simulink model "master_thesis_simulink"  (R2022a)
settings: Solver=VariableStepAuto  StartTime=0.0  StopTime=p_0p.time(end)  FixedStep=0.001  RelTol=1e-3
values from neighbouring files (symbols this model uses):
  markers_forearm = [0.00210510253906 -0.143263397217 -0.00798474121094]    [markers_forearm.mat]
  markers_shoulder = [0.010127746582 -0.151647644043 -0.0119686279297]    [markers_shoulder.mat]
undefined symbols (not defined in the file or in its folder): arm, DiscIntNeverNeededParam, Discrete, ekf, kf, LS, m, markers_hand, n, noise, q0, q0_LS, q0_model, sample_Time, selected, state_observer, Time, tSh_0_0Conf, X, Y, Z
libraries: sm_lib x2029, nesl_utility x1553, robotlib x75, ctrlSharedLib x8
(part 3 of 70)

== system master_thesis_simulink/Ros2Matlab/S0_F1_H2/Position_M0 & velocity_M0 computation ==
  p_W : Inport
  v_W : Inport  Port=2
  quat_02W : Inport  Port=3
  " " : Subsystem  TreatAsAtomicUnit=on
  If1 : If
  MATLAB Function3 : MATLAB Function  TreatAsAtomicUnit=on
  Scope10 : Scope
  Terminator3 : Terminator
  p_0' : Outport
  v_0' : Outport  Port=2
  tag scope: isNew=global
  wires:
  v_W/1 -> " "/2(v_W)
  quat_02W/1 -> " "/3(quat_02W)
  p_W/1 -> " "/1(p_W)
  If1/1 -> " "/Action
  MATLAB Function3/1(y) -> [isNew], Scope10/1, If1/1
  [M0_isNew] -> MATLAB Function3/1(M0_isNew)
  If1/2 -> Terminator3/1
  " "/1(p_0') -> p_0'/1
  " "/2(v_0') -> v_0'/1
  [M2_isNew] -> MATLAB Function3/2(M2_isNew)
  [M3_isNew] -> MATLAB Function3/3(M3_isNew)
  [M4_isNew] -> MATLAB Function3/4(M4_isNew)

== system master_thesis_simulink/Ros2Matlab/S0_F1_H2/Subscriber ==
  M0 : Subsystem
  M2 : Subsystem
  M3 : Subsystem
  M4 : Subsystem
  Shoulder_RF : Subsystem
  Terminator : Terminator
  p0_W : Outport
  p2_W : Outport  Port=2
  p3_W : Outport  Port=3
  p4_W : Outport  Port=4
  v0_W : Outport  Port=5
  v2_W : Outport  Port=6
  v3_W : Outport  Port=7
  v4_W : Outport  Port=8
  quat_02W : Outport  Port=9
  pSh_W : Outport  Port=10
  Rp0_W : Outport  Port=11
  Rp2_W : Outport  Port=12
  Rp3_W : Outport  Port=13
  Rp4_W : Outport  Port=14
  Rv0_W : Outport  Port=15
  Rv2_W : Outport  Port=16
  Rv3_W : Outport  Port=17
  Rv4_W : Outport  Port=18
  wires:
  M4/2(v4_W) -> v4_W/1  "v4_W"
  M2/1(p2_W) -> p2_W/1  "p2_W"
  M2/2(v2_W) -> v2_W/1  "v2_W"
  Shoulder_RF/1(pSh_W) -> pSh_W/1
  M0/2(v0_W) -> v0_W/1  "v0_W"
  M3/1(p3_W) -> p3_W/1  "p3_W"
  M3/2(v3_W) -> v3_W/1  "v3_W"
  M0/3(quat_02W) -> quat_02W/1
  M0/1(p0_W) -> p0_W/1  "p0_W"
  M4/1(p4_W) -> p4_W/1  "p4_W"
  Shoulder_RF/2(quat_Sh2W) -> Terminator/1
  M0/4(Rp0_W) -> Rp0_W/1  "Covariance Rp0_W"
  M2/3(Rp2_W) -> Rp2_W/1  "Covariance Rp2_W"
  M3/3(Rp3_W) -> Rp3_W/1  "Covariance Rp3_W"
  M4/3(Rp4_W) -> Rp4_W/1  "Covariance Rp4_W"
  M0/5(Rv0_W) -> Rv0_W/1  "Covariance Rv0_W"
  M2/4(Rv2_W) -> Rv2_W/1  "Covariance Rv2_W"
  M3/4(Rv3_W) -> Rv3_W/1  "Covariance Rv3_W"
  M4/4(Rv4_W) -> Rv4_W/1  "Covariance Rv4_W"

== system master_thesis_simulink/Ros2Matlab/S0_F1_H2/tSh_0 computation ==
  p0_W : Inport
  pSh_W : Inport  Port=2
  quat_02W : Inport  Port=3
  If Action Subsystem1 : Subsystem  TreatAsAtomicUnit=on
  If1 : If
  MATLAB Function3 : MATLAB Function  TreatAsAtomicUnit=on
  Scope10 : Scope
  Terminator3 : Terminator
  tSh_0 : Outport
  wires:
  [Sh_isNew] -> MATLAB Function3/2(Sh_isNew)
  If1/2 -> Terminator3/1
  If Action Subsystem1/1(tSh_0) -> tSh_0/1
  [M0_isNew] -> MATLAB Function3/1(M0_isNew)
  p0_W/1 -> If Action Subsystem1/1(p0_W)
  MATLAB Function3/1(y) -> Scope10/1, If1/1
  If1/1 -> If Action Subsystem1/Action
  pSh_W/1 -> If Action Subsystem1/2(pSh_W)
  quat_02W/1 -> If Action Subsystem1/3(quat_02W)

== system master_thesis_simulink/Ros2Matlab/S0_F2_H2/Position_M0 & velocity_M0 computation ==
  p_W : Inport
  v_W : Inport  Port=2
  quat_02W : Inport  Port=3
  " " : Subsystem  TreatAsAtomicUnit=on
  If1 : If
  MATLAB Function3 : MATLAB Function  TreatAsAtomicUnit=on
  Scope10 : Scope
  Terminator3 : Terminator
  p_0' : Outport
  v_0' : Outport  Port=2
  tag scope: isNew=global
  wires:
  v_W/1 -> " "/2(v_W)
  quat_02W/1 -> " "/3(quat_02W)
  p_W/1 -> " "/1(p_W)
  If1/1 -> " "/Action
  [M1_isNew] -> MATLAB Function3/2(M1_isNew)
  MATLAB Function3/1(y) -> [isNew], Scope10/1, If1/1
  [M0_isNew] -> MATLAB Function3/1(M0_isNew)
  If1/2 -> Terminator3/1
  " "/1(p_0') -> p_0'/1
  " "/2(v_0') -> v_0'/1
  [M2_isNew] -> MATLAB Function3/3(M2_isNew)
  [M3_isNew] -> MATLAB Function3/4(M3_isNew)
  [M4_isNew] -> MATLAB Function3/5(M4_isNew)

== system master_thesis_simulink/Ros2Matlab/S0_F2_H2/Subscriber ==
  M0 : Subsystem
  M1 : Subsystem
  M2 : Subsystem
  M3 : Subsystem
  M4 : Subsystem
  Shoulder_RF : Subsystem
  Terminator : Terminator
  p0_W : Outport
  p1_W : Outport  Port=2
  p2_W : Outport  Port=3
  p3_W : Outport  Port=4
  p4_W : Outport  Port=5
  v0_W : Outport  Port=6
  v1_W : Outport  Port=7
  v2_W : Outport  Port=8
  v3_W : Outport  Port=9
  v4_W : Outport  Port=10
  quat_02W : Outport  Port=11
  pSh_W : Outport  Port=12
  Rp0_W : Outport  Port=13
  Rp1_W : Outport  Port=14
  Rp2_W : Outport  Port=15
  Rp3_W : Outport  Port=16
  Rp4_W : Outport  Port=17
  Rv0_W : Outport  Port=18
  Rv1_W : Outport  Port=19
  Rv2_W : Outport  Port=20
  Rv3_W : Outport  Port=21
  Rv4_W : Outport  Port=22
  wires:
  M4/2(v4_W) -> v4_W/1  "v4_W"
  M2/1(p2_W) -> p2_W/1  "p2_W"
  M2/2(v2_W) -> v2_W/1  "v2_W"
  Shoulder_RF/1(pSh_W) -> pSh_W/1
  M1/1(p1_W) -> p1_W/1  "p1_W"
  M0/2(v0_W) -> v0_W/1  "v0_W"
  M3/1(p3_W) -> p3_W/1  "p3_W"
  M3/2(v3_W) -> v3_W/1  "v3_W"
  M0/3(quat_02W) -> quat_02W/1
  M0/1(p0_W) -> p0_W/1  "p0_W"
  M1/2(v1_W) -> v1_W/1  "v1_W"
  M4/1(p4_W) -> p4_W/1  "p4_W"
  Shoulder_RF/2(quat_Sh2W) -> Terminator/1
  M0/4(Rp0_W) -> Rp0_W/1  "Covariance Rp0_W"
  M1/3(Rp1_W) -> Rp1_W/1  "Covariance Rp1_W"
  M2/3(Rp2_W) -> Rp2_W/1  "Covariance Rp2_W"
  M3/3(Rp3_W) -> Rp3_W/1  "Covariance Rp3_W"
  M4/3(Rp4_W) -> Rp4_W/1  "Covariance Rp4_W"
  M0/5(Rv0_W) -> Rv0_W/1  "Covariance Rv0_W"
  M1/4(Rv1_W) -> Rv1_W/1  "Covariance Rv1_W"
  M2/4(Rv2_W) -> Rv2_W/1  "Covariance Rv2_W"
  M3/4(Rv3_W) -> Rv3_W/1  "Covariance Rv3_W"
  M4/4(Rv4_W) -> Rv4_W/1  "Covariance Rv4_W"

== system master_thesis_simulink/Ros2Matlab/S0_F2_H2/tSh_0 computation ==
  p0_W : Inport
  pSh_W : Inport  Port=2
  quat_02W : Inport  Port=3
  If Action Subsystem1 : Subsystem  TreatAsAtomicUnit=on
  If1 : If
  MATLAB Function3 : MATLAB Function  TreatAsAtomicUnit=on
  Scope10 : Scope
  Terminator3 : Terminator
  tSh_0 : Outport
  wires:
  [Sh_isNew] -> MATLAB Function3/2(Sh_isNew)
  If1/2 -> Terminator3/1
  If Action Subsystem1/1(tSh_0) -> tSh_0/1
  [M0_isNew] -> MATLAB Function3/1(M0_isNew)
  p0_W/1 -> If Action Subsystem1/1(p0_W)
  MATLAB Function3/1(y) -> Scope10/1, If1/1
  If1/1 -> If Action Subsystem1/Action
  pSh_W/1 -> If Action Subsystem1/2(pSh_W)
  quat_02W/1 -> If Action Subsystem1/3(quat_02W)

== system master_thesis_simulink/Ros2Matlab/S1_F0_H2/Position_M0 & velocity_M0 computation ==
  p_W : Inport
  v_W : Inport  Port=2
  quat_02W : Inport  Port=3
  " " : Subsystem  TreatAsAtomicUnit=on
  If1 : If
  MATLAB Function3 : MATLAB Function  TreatAsAtomicUnit=on
  Scope10 : Scope
  Terminator3 : Terminator
  p_0' : Outport
  v_0' : Outport  Port=2
  tag scope: isNew=global
  wires:
  v_W/1 -> " "/2(v_W)
  quat_02W/1 -> " "/3(quat_02W)
  p_W/1 -> " "/1(p_W)
  If1/1 -> " "/Action
  [M1_isNew] -> MATLAB Function3/2(M1_isNew)
  MATLAB Function3/1(y) -> [isNew], Scope10/1, If1/1
  [M0_isNew] -> MATLAB Function3/1(M0_isNew)
  If1/2 -> Terminator3/1
  " "/1(p_0') -> p_0'/1
  " "/2(v_0') -> v_0'/1
  [M3_isNew] -> MATLAB Function3/3(M3_isNew)
  [M4_isNew] -> MATLAB Function3/4(M4_isNew)

== system master_thesis_simulink/Ros2Matlab/S1_F0_H2/Subscriber ==
  M0 : Subsystem
  M1 : Subsystem
  M3 : Subsystem
  M4 : Subsystem
  Shoulder_RF : Subsystem
  Terminator : Terminator
  p0_W : Outport
  p1_W : Outport  Port=2
  p3_W : Outport  Port=3
  p4_W : Outport  Port=4
  v0_W : Outport  Port=5
  v1_W : Outport  Port=6
  v3_W : Outport  Port=7
  v4_W : Outport  Port=8
  quat_02W : Outport  Port=9
  pSh_W : Outport  Port=10
  Rp0_W : Outport  Port=11
  Rp1_W : Outport  Port=12
  Rp3_W : Outport  Port=13
  Rp4_W : Outport  Port=14
  Rv0_W : Outport  Port=15
  Rv1_W : Outport  Port=16
  Rv3_W : Outport  Port=17
  Rv4_W : Outport  Port=18
  wires:
  M4/2(v4_W) -> v4_W/1  "v4_W"
  Shoulder_RF/1(pSh_W) -> pSh_W/1
  M1/1(p1_W) -> p1_W/1  "p1_W"
  M0/2(v0_W) -> v0_W/1  "v0_W"
  M3/1(p3_W) -> p3_W/1  "p3_W"
  M3/2(v3_W) -> v3_W/1  "v3_W"
  M0/3(quat_02W) -> quat_02W/1
  M0/1(p0_W) -> p0_W/1  "p0_W"
  M1/2(v1_W) -> v1_W/1  "v1_W"
  M4/1(p4_W) -> p4_W/1  "p4_W"
  Shoulder_RF/2(quat_Sh2W) -> Terminator/1
  M0/4(Rp0_W) -> Rp0_W/1  "Covariance Rp0_W"
  M1/3(Rp1_W) -> Rp1_W/1  "Covariance Rp1_W"
  M3/3(Rp3_W) -> Rp3_W/1  "Covariance Rp3_W"
  M4/3(Rp4_W) -> Rp4_W/1  "Covariance Rp4_W"
  M0/5(Rv0_W) -> Rv0_W/1  "Covariance Rv0_W"
  M1/4(Rv1_W) -> Rv1_W/1  "Covariance Rv1_W"
  M3/4(Rv3_W) -> Rv3_W/1  "Covariance Rv3_W"
  M4/4(Rv4_W) -> Rv4_W/1  "Covariance Rv4_W"

== system master_thesis_simulink/Ros2Matlab/S1_F0_H2/tSh_0 computation ==
  p0_W : Inport
  pSh_W : Inport  Port=2
  quat_02W : Inport  Port=3
  If Action Subsystem1 : Subsystem  TreatAsAtomicUnit=on
  If1 : If
  MATLAB Function3 : MATLAB Function  TreatAsAtomicUnit=on
  Scope10 : Scope
  Terminator3 : Terminator
  tSh_0 : Outport
  wires:
  [Sh_isNew] -> MATLAB Function3/2(Sh_isNew)
  If1/2 -> Terminator3/1
  If Action Subsystem1/1(tSh_0) -> tSh_0/1
  [M0_isNew] -> MATLAB Function3/1(M0_isNew)
  p0_W/1 -> If Action Subsystem1/1(p0_W)
  MATLAB Function3/1(y) -> Scope10/1, If1/1
  If1/1 -> If Action Subsystem1/Action
  pSh_W/1 -> If Action Subsystem1/2(pSh_W)
  quat_02W/1 -> If Action Subsystem1/3(quat_02W)

== system master_thesis_simulink/Ros2Matlab/S1_F0_H3/Position_M0 & velocity_M0 computation ==
  p_W : Inport
  v_W : Inport  Port=2
  quat_02W : Inport  Port=3
  " " : Subsystem  TreatAsAtomicUnit=on
  If1 : If
  MATLAB Function3 : MATLAB Function  TreatAsAtomicUnit=on
  Scope10 : Scope
  Terminator3 : Terminator
  p_0' : Outport
  v_0' : Outport  Port=2
  tag scope: isNew=global
  wires:
  v_W/1 -> " "/2(v_W)
  quat_02W/1 -> " "/3(quat_02W)
  p_W/1 -> " "/1(p_W)
  If1/1 -> " "/Action
  [M1_isNew] -> MATLAB Function3/2(M1_isNew)
  MATLAB Function3/1(y) -> [isNew], Scope10/1, If1/1
  [M0_isNew] -> MATLAB Function3/1(M0_isNew)
  If1/2 -> Terminator3/1
  " "/1(p_0') -> p_0'/1
  " "/2(v_0') -> v_0'/1
  [M2_isNew] -> MATLAB Function3/3(M2_isNew)
  [M3_isNew] -> MATLAB Function3/4(M3_isNew)
  [M4_isNew] -> MATLAB Function3/5(M4_isNew)

== system master_thesis_simulink/Ros2Matlab/S1_F0_H3/Subscriber ==
  M0 : Subsystem
  M1 : Subsystem
  M2 : Subsystem
  M3 : Subsystem
  M4 : Subsystem
  Shoulder_RF : Subsystem
  Terminator : Terminator
  p0_W : Outport
  p1_W : Outport  Port=2
  p2_W : Outport  Port=3
  p3_W : Outport  Port=4
  p4_W : Outport  Port=5
  v0_W : Outport  Port=6
  v1_W : Outport  Port=7
  v2_W : Outport  Port=8
  v3_W : Outport  Port=9
  v4_W : Outport  Port=10
  quat_02W : Outport  Port=11
  pSh_W : Outport  Port=12
  Rp0_W : Outport  Port=13
  Rp1_W : Outport  Port=14
  Rp2_W : Outport  Port=15
  Rp3_W : Outport  Port=16
  Rp4_W : Outport  Port=17
  Rv0_W : Outport  Port=18
  Rv1_W : Outport  Port=19
  Rv2_W : Outport  Port=20
  Rv3_W : Outport  Port=21
  Rv4_W : Outport  Port=22
  wires:
  M4/2(v4_W) -> v4_W/1  "v4_W"
  M2/1(p2_W) -> p2_W/1  "p2_W"
  M2/2(v2_W) -> v2_W/1  "v2_W"
  Shoulder_RF/1(pSh_W) -> pSh_W/1
  M1/1(p1_W) -> p1_W/1  "p1_W"
  M0/2(v0_W) -> v0_W/1  "v0_W"
  M3/1(p3_W) -> p3_W/1  "p3_W"
  M3/2(v3_W) -> v3_W/1  "v3_W"
  M0/3(quat_02W) -> quat_02W/1
  M0/1(p0_W) -> p0_W/1  "p0_W"
  M1/2(v1_W) -> v1_W/1  "v1_W"
  M4/1(p4_W) -> p4_W/1  "p4_W"
  Shoulder_RF/2(quat_Sh2W) -> Terminator/1
  M0/4(Rp0_W) -> Rp0_W/1  "Covariance Rp0_W"
  M1/3(Rp1_W) -> Rp1_W/1  "Covariance Rp1_W"
  M2/3(Rp2_W) -> Rp2_W/1  "Covariance Rp2_W"
  M3/3(Rp3_W) -> Rp3_W/1  "Covariance Rp3_W"
  M4/3(Rp4_W) -> Rp4_W/1  "Covariance Rp4_W"
  M0/5(Rv0_W) -> Rv0_W/1  "Covariance Rv0_W"
  M1/4(Rv1_W) -> Rv1_W/1  "Covariance Rv1_W"
  M2/4(Rv2_W) -> Rv2_W/1  "Covariance Rv2_W"
  M3/4(Rv3_W) -> Rv3_W/1  "Covariance Rv3_W"
  M4/4(Rv4_W) -> Rv4_W/1  "Covariance Rv4_W"

== system master_thesis_simulink/Ros2Matlab/S1_F0_H3/tSh_0 computation ==
  p0_W : Inport
  pSh_W : Inport  Port=2
  quat_02W : Inport  Port=3
  If Action Subsystem1 : Subsystem  TreatAsAtomicUnit=on
  If1 : If
  MATLAB Function3 : MATLAB Function  TreatAsAtomicUnit=on
  Scope10 : Scope
  Terminator3 : Terminator
  tSh_0 : Outport
  wires:
  [Sh_isNew] -> MATLAB Function3/2(Sh_isNew)
  If1/2 -> Terminator3/1
  If Action Subsystem1/1(tSh_0) -> tSh_0/1
  [M0_isNew] -> MATLAB Function3/1(M0_isNew)
  p0_W/1 -> If Action Subsystem1/1(p0_W)
  MATLAB Function3/1(y) -> Scope10/1, If1/1
  If1/1 -> If Action Subsystem1/Action
  pSh_W/1 -> If Action Subsystem1/2(pSh_W)
  quat_02W/1 -> If Action Subsystem1/3(quat_02W)

== system master_thesis_simulink/Ros2Matlab/S1_F1_H2/Position_M0 & velocity_M0 computation ==
  p_W : Inport
  v_W : Inport  Port=2
  quat_02W : Inport  Port=3
  " " : Subsystem  TreatAsAtomicUnit=on
  If1 : If
  MATLAB Function3 : MATLAB Function  TreatAsAtomicUnit=on
  Scope10 : Scope
  Terminator3 : Terminator
  p_0' : Outport
  v_0' : Outport  Port=2
  tag scope: isNew=global
  wires:
  v_W/1 -> " "/2(v_W)
  quat_02W/1 -> " "/3(quat_02W)
  p_W/1 -> " "/1(p_W)
  If1/1 -> " "/Action
  [M1_isNew] -> MATLAB Function3/2(M1_isNew)
  MATLAB Function3/1(y) -> [isNew], Scope10/1, If1/1
  [M0_isNew] -> MATLAB Function3/1(M0_isNew)
  If1/2 -> Terminator3/1
  " "/1(p_0') -> p_0'/1
  " "/2(v_0') -> v_0'/1
  [M2_isNew] -> MATLAB Function3/3(M2_isNew)
  [M3_isNew] -> MATLAB Function3/4(M3_isNew)
  [M4_isNew] -> MATLAB Function3/5(M4_isNew)

== system master_thesis_simulink/Ros2Matlab/S1_F1_H2/Subscriber ==
  M0 : Subsystem
  M1 : Subsystem
  M2 : Subsystem
  M3 : Subsystem
  M4 : Subsystem
  Shoulder_RF : Subsystem
  Terminator : Terminator
  p0_W : Outport
  p1_W : Outport  Port=2
  p2_W : Outport  Port=3
  p3_W : Outport  Port=4
  p4_W : Outport  Port=5
  v0_W : Outport  Port=6
  v1_W : Outport  Port=7
  v2_W : Outport  Port=8
  v3_W : Outport  Port=9
  v4_W : Outport  Port=10
  quat_02W : Outport  Port=11
  pSh_W : Outport  Port=12
  Rp0_W : Outport  Port=13
  Rp1_W : Outport  Port=14
  Rp2_W : Outport  Port=15
  Rp3_W : Outport  Port=16
  Rp4_W : Outport  Port=17
  Rv0_W : Outport  Port=18
  Rv1_W : Outport  Port=19
  Rv2_W : Outport  Port=20
  Rv3_W : Outport  Port=21
  Rv4_W : Outport  Port=22
  wires:
  M4/2(v4_W) -> v4_W/1  "v4_W"
  M2/1(p2_W) -> p2_W/1  "p2_W"
  M2/2(v2_W) -> v2_W/1  "v2_W"
  Shoulder_RF/1(pSh_W) -> pSh_W/1
  M1/1(p1_W) -> p1_W/1  "p1_W"
  M0/2(v0_W) -> v0_W/1  "v0_W"
  M3/1(p3_W) -> p3_W/1  "p3_W"
  M3/2(v3_W) -> v3_W/1  "v3_W"
  M0/3(quat_02W) -> quat_02W/1
  M0/1(p0_W) -> p0_W/1  "p0_W"
  M1/2(v1_W) -> v1_W/1  "v1_W"
  M4/1(p4_W) -> p4_W/1  "p4_W"
  Shoulder_RF/2(quat_Sh2W) -> Terminator/1
  M0/4(Rp0_W) -> Rp0_W/1  "Covariance Rp0_W"
  M1/3(Rp1_W) -> Rp1_W/1  "Covariance Rp1_W"
  M2/3(Rp2_W) -> Rp2_W/1  "Covariance Rp2_W"
  M3/3(Rp3_W) -> Rp3_W/1  "Covariance Rp3_W"
  M4/3(Rp4_W) -> Rp4_W/1  "Covariance Rp4_W"
  M0/5(Rv0_W) -> Rv0_W/1  "Covariance Rv0_W"
  M1/4(Rv1_W) -> Rv1_W/1  "Covariance Rv1_W"
  M2/4(Rv2_W) -> Rv2_W/1  "Covariance Rv2_W"
  M3/4(Rv3_W) -> Rv3_W/1  "Covariance Rv3_W"
  M4/4(Rv4_W) -> Rv4_W/1  "Covariance Rv4_W"

== system master_thesis_simulink/Ros2Matlab/S1_F1_H2/tSh_0 computation ==
  p0_W : Inport
  pSh_W : Inport  Port=2
  quat_02W : Inport  Port=3
  If Action Subsystem1 : Subsystem  TreatAsAtomicUnit=on
  If1 : If
  MATLAB Function3 : MATLAB Function  TreatAsAtomicUnit=on
  Scope10 : Scope
  Terminator3 : Terminator
  tSh_0 : Outport
  wires:
  [Sh_isNew] -> MATLAB Function3/2(Sh_isNew)
  If1/2 -> Terminator3/1
  If Action Subsystem1/1(tSh_0) -> tSh_0/1
  [M0_isNew] -> MATLAB Function3/1(M0_isNew)
  p0_W/1 -> If Action Subsystem1/1(p0_W)
  MATLAB Function3/1(y) -> Scope10/1, If1/1
  If1/1 -> If Action Subsystem1/Action
  pSh_W/1 -> If Action Subsystem1/2(pSh_W)
  quat_02W/1 -> If Action Subsystem1/3(quat_02W)

== system master_thesis_simulink/Ros2Matlab/S1_F2_H2/Position_M0 & velocity_M0 computation ==
  p_W : Inport
  v_W : Inport  Port=2
  quat_02W : Inport  Port=3
  " " : Subsystem  TreatAsAtomicUnit=on
  If1 : If
  MATLAB Function3 : MATLAB Function  TreatAsAtomicUnit=on
  Scope10 : Scope
  Terminator3 : Terminator
  p_0' : Outport
  v_0' : Outport  Port=2
  tag scope: isNew=global
  wires:
  [M4_isNew] -> MATLAB Function3/5(M4_isNew)
  [M3_isNew] -> MATLAB Function3/4(M3_isNew)
  [M2_isNew] -> MATLAB Function3/3(M2_isNew)
  " "/2(v_0') -> v_0'/1
  " "/1(p_0') -> p_0'/1
  If1/2 -> Terminator3/1
  [M0_isNew] -> MATLAB Function3/1(M0_isNew)
  MATLAB Function3/1(y) -> If1/1, Scope10/1, [isNew]
  [M1_isNew] -> MATLAB Function3/2(M1_isNew)
  If1/1 -> " "/Action
  p_W/1 -> " "/1(p_W)
  quat_02W/1 -> " "/3(quat_02W)
  v_W/1 -> " "/2(v_W)
  [M5_isNew] -> MATLAB Function3/6(M5_isNew)

== system master_thesis_simulink/Ros2Matlab/S1_F2_H2/Subscriber ==
  M0 : Subsystem
  M1 : Subsystem
  M2 : Subsystem
  M3 : Subsystem
  M4 : Subsystem
  M5 : Subsystem
  Shoulder_RF : Subsystem
  Terminator : Terminator
  p0_W : Outport
  p1_W : Outport  Port=2
  p2_W : Outport  Port=3
  p3_W : Outport  Port=4
  p4_W : Outport  Port=5
  v0_W : Outport  Port=6
  v1_W : Outport  Port=7
  v2_W : Outport  Port=8
  v3_W : Outport  Port=9
  v4_W : Outport  Port=10
  quat_02W : Outport  Port=11
  pSh_W : Outport  Port=12
  Rp0_W : Outport  Port=13
  Rp1_W : Outport  Port=14
  Rp2_W : Outport  Port=15
  Rp3_W : Outport  Port=16
  Rp4_W : Outport  Port=17
  Rv0_W : Outport  Port=18
  Rv1_W : Outport  Port=19
  Rv2_W : Outport  Port=20
  Rv3_W : Outport  Port=21
  Rv4_W : Outport  Port=22
  p5_W : Outport  Port=23
  v5_W : Outport  Port=24
  Rp5_W : Outport  Port=25
  Rv5_W : Outport  Port=26
  wires:
  M4/4(Rv4_W) -> Rv4_W/1  "Covariance Rv4_W"
  M3/4(Rv3_W) -> Rv3_W/1  "Covariance Rv3_W"
  M2/4(Rv2_W) -> Rv2_W/1  "Covariance Rv2_W"
  M1/4(Rv1_W) -> Rv1_W/1  "Covariance Rv1_W"
  M0/5(Rv0_W) -> Rv0_W/1  "Covariance Rv0_W"
  M4/3(Rp4_W) -> Rp4_W/1  "Covariance Rp4_W"
  M3/3(Rp3_W) -> Rp3_W/1  "Covariance Rp3_W"
  M2/3(Rp2_W) -> Rp2_W/1  "Covariance Rp2_W"
  M1/3(Rp1_W) -> Rp1_W/1  "Covariance Rp1_W"
  M0/4(Rp0_W) -> Rp0_W/1  "Covariance Rp0_W"
  Shoulder_RF/2(quat_Sh2W) -> Terminator/1
  M4/1(p4_W) -> p4_W/1  "p4_W"
  M1/2(v1_W) -> v1_W/1  "v1_W"
  M0/1(p0_W) -> p0_W/1  "p0_W"
  M0/3(quat_02W) -> quat_02W/1
  M3/2(v3_W) -> v3_W/1  "v3_W"
  M3/1(p3_W) -> p3_W/1  "p3_W"
  M0/2(v0_W) -> v0_W/1  "v0_W"
  M1/1(p1_W) -> p1_W/1  "p1_W"
  Shoulder_RF/1(pSh_W) -> pSh_W/1
  M2/2(v2_W) -> v2_W/1  "v2_W"
  M2/1(p2_W) -> p2_W/1  "p2_W"
  M4/2(v4_W) -> v4_W/1  "v4_W"
  M5/1(p2_W) -> p5_W/1  "p2_W"
  M5/2(v2_W) -> v5_W/1  "v2_W"
  M5/3(Rp2_W) -> Rp5_W/1  "Covariance Rp2_W"
  M5/4(Rv2_W) -> Rv5_W/1  "Covariance Rv2_W"

== system master_thesis_simulink/Ros2Matlab/S1_F2_H2/tSh_0 computation ==
  p0_W : Inport
  pSh_W : Inport  Port=2
  quat_02W : Inport  Port=3
  If Action Subsystem1 : Subsystem  TreatAsAtomicUnit=on
  If1 : If
  MATLAB Function3 : MATLAB Function  TreatAsAtomicUnit=on
  Scope10 : Scope
  Terminator3 : Terminator
  tSh_0 : Outport
  wires:
  quat_02W/1 -> If Action Subsystem1/3(quat_02W)
  pSh_W/1 -> If Action Subsystem1/2(pSh_W)
  If1/1 -> If Action Subsystem1/Action
  MATLAB Function3/1(y) -> If1/1, Scope10/1
  p0_W/1 -> If Action Subsystem1/1(p0_W)
  [M0_isNew] -> MATLAB Function3/1(M0_isNew)
  If Action Subsystem1/1(tSh_0) -> tSh_0/1
  If1/2 -> Terminator3/1
  [Sh_isNew] -> MATLAB Function3/2(Sh_isNew)

== system master_thesis_simulink/Ros2Matlab/S2_F0_H2/Position_M0 & velocity_M0 computation ==
  p_W : Inport
  v_W : Inport  Port=2
  quat_02W : Inport  Port=3
  " " : Subsystem  TreatAsAtomicUnit=on
  If1 : If
  MATLAB Function3 : MATLAB Function  TreatAsAtomicUnit=on
  Scope10 : Scope
  Terminator3 : Terminator
  p_0' : Outport
  v_0' : Outport  Port=2
  tag scope: isNew=global
  wires:
  v_W/1 -> " "/2(v_W)
  quat_02W/1 -> " "/3(quat_02W)
  p_W/1 -> " "/1(p_W)
  If1/1 -> " "/Action
  [M1_isNew] -> MATLAB Function3/2(M1_isNew)
  MATLAB Function3/1(y) -> [isNew], Scope10/1, If1/1
  [M0_isNew] -> MATLAB Function3/1(M0_isNew)
  If1/2 -> Terminator3/1
  " "/1(p_0') -> p_0'/1
  " "/2(v_0') -> v_0'/1
  [M2_isNew] -> MATLAB Function3/3(M2_isNew)
  [M3_isNew] -> MATLAB Function3/4(M3_isNew)
  [M4_isNew] -> MATLAB Function3/5(M4_isNew)

== system master_thesis_simulink/Ros2Matlab/S2_F0_H2/Subscriber ==
  M0 : Subsystem
  M1 : Subsystem
  M2 : Subsystem
  M3 : Subsystem
  M4 : Subsystem
  Shoulder_RF : Subsystem
  Terminator : Terminator
  p0_W : Outport
  p1_W : Outport  Port=2
  p2_W : Outport  Port=3
  p3_W : Outport  Port=4
  p4_W : Outport  Port=5
  v0_W : Outport  Port=6
  v1_W : Outport  Port=7
  v2_W : Outport  Port=8
  v3_W : Outport  Port=9
  v4_W : Outport  Port=10
  quat_02W : Outport  Port=11
  pSh_W : Outport  Port=12
  Rp0_W : Outport  Port=13
  Rp1_W : Outport  Port=14
  Rp2_W : Outport  Port=15
  Rp3_W : Outport  Port=16
  Rp4_W : Outport  Port=17
  Rv0_W : Outport  Port=18
  Rv1_W : Outport  Port=19
  Rv2_W : Outport  Port=20
  Rv3_W : Outport  Port=21
  Rv4_W : Outport  Port=22
  wires:
  M4/2(v4_W) -> v4_W/1  "v4_W"
  M2/1(p2_W) -> p2_W/1  "p2_W"
  M2/2(v2_W) -> v2_W/1  "v2_W"
  Shoulder_RF/1(pSh_W) -> pSh_W/1
  M1/1(p1_W) -> p1_W/1  "p1_W"
  M0/2(v0_W) -> v0_W/1  "v0_W"
  M3/1(p3_W) -> p3_W/1  "p3_W"
  M3/2(v3_W) -> v3_W/1  "v3_W"
  M0/3(quat_02W) -> quat_02W/1
  M0/1(p0_W) -> p0_W/1  "p0_W"
  M1/2(v1_W) -> v1_W/1  "v1_W"
  M4/1(p4_W) -> p4_W/1  "p4_W"
  Shoulder_RF/2(quat_Sh2W) -> Terminator/1
  M0/4(Rp0_W) -> Rp0_W/1  "Covariance Rp0_W"
  M1/3(Rp1_W) -> Rp1_W/1  "Covariance Rp1_W"
  M2/3(Rp2_W) -> Rp2_W/1  "Covariance Rp2_W"
  M3/3(Rp3_W) -> Rp3_W/1  "Covariance Rp3_W"
  M4/3(Rp4_W) -> Rp4_W/1  "Covariance Rp4_W"
  M0/5(Rv0_W) -> Rv0_W/1  "Covariance Rv0_W"
  M1/4(Rv1_W) -> Rv1_W/1  "Covariance Rv1_W"
  M2/4(Rv2_W) -> Rv2_W/1  "Covariance Rv2_W"
  M3/4(Rv3_W) -> Rv3_W/1  "Covariance Rv3_W"
  M4/4(Rv4_W) -> Rv4_W/1  "Covariance Rv4_W"

== system master_thesis_simulink/Ros2Matlab/S2_F0_H2/tSh_0 computation ==
  p0_W : Inport
  pSh_W : Inport  Port=2
  quat_02W : Inport  Port=3
  If Action Subsystem1 : Subsystem  TreatAsAtomicUnit=on
  If1 : If
  MATLAB Function3 : MATLAB Function  TreatAsAtomicUnit=on
  Scope10 : Scope
  Terminator3 : Terminator
  tSh_0 : Outport
  wires:
  [Sh_isNew] -> MATLAB Function3/2(Sh_isNew)
  If1/2 -> Terminator3/1
  If Action Subsystem1/1(tSh_0) -> tSh_0/1
  [M0_isNew] -> MATLAB Function3/1(M0_isNew)
  p0_W/1 -> If Action Subsystem1/1(p0_W)
  MATLAB Function3/1(y) -> Scope10/1, If1/1
  If1/1 -> If Action Subsystem1/Action
  pSh_W/1 -> If Action Subsystem1/2(pSh_W)
  quat_02W/1 -> If Action Subsystem1/3(quat_02W)

== system master_thesis_simulink/System/Human arm/Elbow_joint ==
  q ref 4 : Inport
  PS-Simulink Converter1 : nesl_utility/PS-Simulink Converter  PhysicalDomain=network_engine_domain  SubClassName=ps_output  LeftPortType=input  RightPortType=output  PseudoPeriodic=off  Frequencies=[]  VectorFormat=inherit  Unit=inherit  AffineConversion=off
      settings: SourceProductBaseCode=SS,PW,VE
  PS-Simulink Converter6 : nesl_utility/PS-Simulink Converter  PhysicalDomain=network_engine_domain  SubClassName=ps_output  LeftPortType=input  RightPortType=output  PseudoPeriodic=off  Frequencies=[]  VectorFormat=inherit  Unit=inherit  AffineConversion=off
      settings: SourceProductBaseCode=SS,PW,VE
  c1 : nesl_utility/Simulink-PS Converter  PhysicalDomain=network_engine_domain  SubClassName=ps_input  LeftPortType=input  RightPortType=output  PseudoPeriodic=off  Frequencies=[]  NoiseDistribution=none  NoiseParameters=[]  Unit=1  AffineConversion=off  FilteringAndDerivatives=filter  SimscapeFilterOrder=2  InputFilterTimeConstant=0.001  UdotUserProvided=0
      settings: SourceProductBaseCode=SS,PW,VE
  jRightElbow_rotx : sm_lib/Joints/Revolute Joint  JointMode=Normal  SenseConstraintForce=off  SenseConstraintForceX=off  SenseConstraintForceY=off  SenseConstraintForceZ=off  SenseConstraintTorque=off  SenseConstraintTorqueX=off  SenseConstraintTorqueY=off  SenseConstraintTorqueZ=off  SenseTotalForce=off  SenseTotalForceX=off  SenseTotalForceY=off  SenseTotalForceZ=off  SenseTotalTorque=off  SenseTotalTorqueX=off  SenseTotalTorqueY=off  SenseTotalTorqueZ=off  CompositeWrenchDir=FollowerOnBase  CompositeWrenchFrame=BaseFrame  EquilibriumPosition=0  EquilibriumPositionUnits=deg  SpringStiffness=0  SpringStiffnessUnits=N*m/deg  DampingCoefficient=0.1  DampingCoefficientUnits=kg*m^2/(rad*s)  TorqueActuationMode=ComputedTorque  MotionActuationMode=InputMotion  SensePosition=on  SenseVelocity=on  SenseAcceleration=off  SenseTorqueForce=off  SenseLowerLimitTorqueForce=off  SenseUpperLimitTorqueForce=off  LowerLimitSpecify=on  LowerLimitBound=-3/4*pi  LowerLimitBoundUnits=rad  LowerLimitStiffness=1e4  LowerLimitStiffnessUnits=N*m/deg  LowerLimitDamping=10  LowerLimitDampingUnits=N*m/(deg/s)  LowerLimitTransitionRegionWidth=0.1  LowerLimitTransitionRegionWidthUnits=deg  UpperLimitSpecify=on  UpperLimitBound=0  UpperLimitBoundUnits=rad  UpperLimitStiffness=1e4  UpperLimitStiffnessUnits=N*m/deg  UpperLimitDamping=10  UpperLimitDampingUnits=N*m/(deg/s)  UpperLimitTransitionRegionWidth=0.1  UpperLimitTransitionRegionWidthUnits=deg  PositionTargetSpecify=off  PositionTargetPriority=High  PositionTargetValue=q0(4)  PositionTargetValueUnits=rad  VelocityTargetSpecify=off  VelocityTargetPriority=High  VelocityTargetValue=0  VelocityTargetValueUnits=deg/s
  B_elbow : PMIOPort  Side=Right
  F_shoulder : PMIOPort  Port=2  Side=Left
  tag scope: q4=global, qdot4=global
  wires:
  PS-Simulink Converter6/1 -> [q4]
  PS-Simulink Converter1/1 -> [qdot4]
  q ref 4/1 -> c1/1
  connections:
  jRightElbow_rotx/RConn2 -- PS-Simulink Converter6/LConn1
  PS-Simulink Converter1/LConn1 -- jRightElbow_rotx/RConn3
  ?
  ?
  F_shoulder/RConn1 -- jRightElbow_rotx/LConn1
  jRightElbow_rotx/RConn1 -- B_elbow/RConn1
  c1/RConn1 -- jRightElbow_rotx/LConn2

== system master_thesis_simulink/System/Human arm/Markers ==
  M1 : Subsystem
  W : PMIOPort  Side=Left
  R : PMIOPort  Port=2  Side=Left
  tag scope: p=global, pdot=global
  wires:
  M1/1(p_1) -> [p]
  M1/2(pdot_1) -> [pdot]
  connections:
  R/RConn1 -- M1/LConn2
  W/RConn1 -- M1/LConn1

== system master_thesis_simulink/System/Human arm/RightForeArm ==
  B_elbow__Eend : sm_lib/Frames and Transforms/Rigid Transform  TranslationMethod=Cartesian  TranslationStandardOffset=0  TranslationLengthUnit=m  TranslationStandardAxis=+Z  TranslationCartesianOffset=[0, -arm.forearm.length, 0]  TranslationROffset=0  TranslationROffsetUnits=m  TranslationZOffset=0  TranslationZOffsetUnits=m  TranslationThetaOffset=0  TranslationThetaOffsetUnits=deg  RotationMethod=None  RotationAngleUnits=deg  RotationStandardAxis=+Z  RotationAngle=0.0  RotationArbitraryAxis=[0 0 1]  FollAlignAxisA=+X  BaseAlignAxisA=+Y  FollAlignAxisB=+Y  BaseAlignAxisB=+Z  RotationSequenceAxes=BaseAxes  RotationSequence=XYZ  RotationSequenceAngles=[0, 0, 0]  RotationSequenceAnglesUnits=rad  RotationMatrix=[1 0 0; 0 1 0; 0 0 1]
  B_elbow_setting : sm_lib/Frames and Transforms/Rigid Transform  TranslationMethod=Cartesian  TranslationStandardOffset=0  TranslationLengthUnit=m  TranslationStandardAxis=+Z  TranslationCartesianOffset=[0, arm.forearm.length/2, 0]  TranslationROffset=0  TranslationROffsetUnits=m  TranslationZOffset=0  TranslationZOffsetUnits=m  TranslationThetaOffset=0  TranslationThetaOffsetUnits=deg  RotationMethod=None  RotationAngleUnits=rad  RotationStandardAxis=+Z  RotationAngle=pi/2  RotationArbitraryAxis=[1 0 0]  FollAlignAxisA=+X  BaseAlignAxisA=+Y  FollAlignAxisB=+Y  BaseAlignAxisB=+Z  RotationSequenceAxes=BaseAxes  RotationSequence=XYZ  RotationSequenceAngles=[pi/2, 0, 0]  RotationSequenceAnglesUnits=rad  RotationMatrix=[1 0 0; 0 1 0; 0 0 1]
  ForeArm : sm_lib/Body Elements/Cylindrical Solid  GraphicAmbientColor=[0.15 0.15 0.15 1.0]  BasedOnType=Density  CenterOfMass=[0, 0, 0]  CenterOfMassUnits=m  GraphicDiffuseColor=[0.1, 0.1, 0.1]  CylinderLength=arm.forearm.length  CylinderLengthUnits=m  CylinderRadius=arm.forearm.radius  CylinderRadiusUnits=m  Density=1000  DensityUnits=kg/m^3  DoExposeReferenceFrame=on  GraphicEmissiveColor=[0.0 0.0 0.0 1.0]  ExportEntireGeometry=off  SerializedFrames=<Frames/>  MarkerShape=Sphere  MarkerSize=10  GraphicType=FromGeometry  InertiaType=CalculateFromGeometry  Mass=0  MassUnits=kg  MomentsOfInertia=[0, 0, 0]  MomentsOfInertiaUnits=kg*m^2  GraphicOpacity=1  ProductsOfInertia=[0, 0, 0]  ProductsOfInertiaUnits=kg*m^2  GraphicShininess=75  GraphicSpecularColor=[0.5 0.5 0.5 1.0]  GraphicVisPropType=SimpleVisualProperties
  Inertia1 : sm_lib/Body Elements/Inertia  InertiaType=Custom  Mass=arm.forearm.mass  MassUnits=kg  CenterOfMass=[0 0 0]  CenterOfMassUnits=m  MomentsOfInertia=arm.forearm.moment_inertia  MomentsOfInertiaUnits=kg*m^2  ProductsOfInertia=[0 0 0]  ProductsOfInertiaUnits=kg*m^2  GraphicType=None  MarkerShape=Inertia  MarkerSize=20  GraphicVisPropType=SimpleVisualProperties  GraphicDiffuseColor=[0.5 0.5 0.5]  GraphicSpecularColor=[0.5 0.5 0.5 1.0]  GraphicAmbientColor=[0.15 0.15 0.15 1.0]  GraphicEmissiveColor=[0.0 0.0 0.0 1.0]  GraphicShininess=75  GraphicOpacity=1.0
  Mux : Mux  Inputs=3
  PS-Simulink Converter : nesl_utility/PS-Simulink Converter  PhysicalDomain=network_engine_domain  SubClassName=ps_output  LeftPortType=input  RightPortType=output  PseudoPeriodic=off  Frequencies=[]  VectorFormat=inherit  Unit=inherit  AffineConversion=off
      settings: SourceProductBaseCode=SS,PW,VE
  PS-Simulink Converter1 : nesl_utility/PS-Simulink Converter  PhysicalDomain=network_engine_domain  SubClassName=ps_output  LeftPortType=input  RightPortType=output  PseudoPeriodic=off  Frequencies=[]  VectorFormat=inherit  Unit=inherit  AffineConversion=off
      settings: SourceProductBaseCode=SS,PW,VE
  PS-Simulink Converter2 : nesl_utility/PS-Simulink Converter  PhysicalDomain=network_engine_domain  SubClassName=ps_output  LeftPortType=input  RightPortType=output  PseudoPeriodic=off  Frequencies=[]  VectorFormat=inherit  Unit=inherit  AffineConversion=off
      settings: SourceProductBaseCode=SS,PW,VE
  Reference Frame : sm_lib/Frames and Transforms/Reference Frame
  RighForeArm_rot : sm_lib/Frames and Transforms/Rigid Transform  TranslationMethod=None  TranslationStandardOffset=0  TranslationLengthUnit=m  TranslationStandardAxis=+Z  TranslationCartesianOffset=[0 0 0]  TranslationROffset=0  TranslationROffsetUnits=m  TranslationZOffset=0  TranslationZOffsetUnits=m  TranslationThetaOffset=0  TranslationThetaOffsetUnits=deg  RotationMethod=ArbitraryAxis  RotationAngleUnits=rad  RotationStandardAxis=+Z  RotationAngle=pi/2  RotationArbitraryAxis=[1 0 0]  FollAlignAxisA=+X  BaseAlignAxisA=+Y  FollAlignAxisB=+Y  BaseAlignAxisB=+Z  RotationSequenceAxes=BaseAxes  RotationSequence=XYZ  RotationSequenceAngles=[pi/2, 0, 0]  RotationSequenceAnglesUnits=rad  RotationMatrix=[1 0 0; 0 1 0; 0 0 1]
  Scope : Scope
  Transform Sensor : sm_lib/Frames and Transforms/Transform Sensor  MeasurementFrame=World  SenseAngle=off  SenseAxis=off  SenseAngle1=off  SenseAngle2=off  SenseAngle3=off  SenseQ=off  SenseR=off  SenseOmegaX=off  SenseOmegaY=off  SenseOmegaZ=off  SenseOmega1=off  SenseOmega2=off  SenseOmega3=off  SenseQDot=off  SenseRDot=off  SenseAlphaX=off  SenseAlphaY=off  SenseAlphaZ=off  SenseAlpha1=off  SenseAlpha2=off  SenseAlpha3=off  SenseQDDot=off  SenseRDDot=off  SenseX=on  SenseY=on  SenseZ=on  SenseRad=off  SenseAzim=off  SenseDist=off  SenseInc=off  SenseXDot=off  SenseYDot=off  SenseZDot=off  SenseRadDot=off  SenseAzimDot=off  SenseDistDot=off  SenseIncDot=off  SenseXDDot=off  SenseYDDot=off  SenseZDDot=off  SenseRadDDot=off  SenseAzimDDot=off  SenseDistDDot=off  SenseIncDDot=off
  B_elbow : PMIOPort  Side=Left
  F_elbow : PMIOPort  Port=2  Side=Right
  W : PMIOPort  Port=3  Side=Left
  wires:
  PS-Simulink Converter2/1 -> Mux/3  "elbow_posz"
  Mux/1 -> Scope/1
  PS-Simulink Converter1/1 -> Mux/2  "elbow_posy"
  PS-Simulink Converter/1 -> Mux/1  "elbow_posx"
  connections:
  B_elbow__Eend/RConn1 -- F_elbow/RConn1
  B_elbow__Eend/LConn1 -- B_elbow_setting/RConn1 -- B_elbow/RConn1 -- Transform Sensor/RConn1
  PS-Simulink Converter/LConn1 -- Transform Sensor/RConn2
  PS-Simulink Converter1/LConn1 -- Transform Sensor/RConn3
  PS-Simulink Converter2/LConn1 -- Transform Sensor/RConn4
  ForeArm/RConn1 -- RighForeArm_rot/LConn1
  W/RConn1 -- Transform Sensor/LConn1
  RighForeArm_rot/RConn1 -- Reference Frame/RConn1 -- Inertia1/RConn1 -- B_elbow_setting/LConn1

== system master_thesis_simulink/System/Human arm/RightHand ==
  B_wrist__setting : sm_lib/Frames and Transforms/Rigid Transform  TranslationMethod=Cartesian  TranslationStandardOffset=0  TranslationLengthUnit=m  TranslationStandardAxis=+Z  TranslationCartesianOffset=[0, arm.hand.dimensions(2)/2, 0]  TranslationROffset=0  TranslationROffsetUnits=m  TranslationZOffset=0  TranslationZOffsetUnits=m  TranslationThetaOffset=0  TranslationThetaOffsetUnits=deg  RotationMethod=None  RotationAngleUnits=deg  RotationStandardAxis=+Z  RotationAngle=0.0  RotationArbitraryAxis=[0 0 1]  FollAlignAxisA=+X  BaseAlignAxisA=+Y  FollAlignAxisB=+Y  BaseAlignAxisB=+Z  RotationSequenceAxes=BaseAxes  RotationSequence=XYZ  RotationSequenceAngles=[0, 0, 0]  RotationSequenceAnglesUnits=rad  RotationMatrix=[1 0 0; 0 1 0; 0 0 1]
  Hand : sm_lib/Body Elements/Brick Solid  GraphicAmbientColor=[0.15 0.15 0.15 1.0]  BasedOnType=Density  BrickDimensions=arm.hand.dimensions  BrickDimensionUnits=m  CenterOfMass=[0, 0, 0]  CenterOfMassUnits=m  GraphicDiffuseColor=[0.1, 0.1, 0.1]  Density=1000  DensityUnits=kg/m^3  DoExposeReferenceFrame=on  GraphicEmissiveColor=[0.0 0.0 0.0 1.0]  ExportEntireGeometry=off  SerializedFrames=<Frames/>  MarkerShape=Sphere  MarkerSize=10  GraphicType=FromGeometry  InertiaType=CalculateFromGeometry  Mass=0  MassUnits=kg  MomentsOfInertia=[0, 0, 0]  MomentsOfInertiaUnits=kg*m^2  GraphicOpacity=1  ProductsOfInertia=[0, 0, 0]  ProductsOfInertiaUnits=kg*m^2  GraphicShininess=75  GraphicSpecularColor=[0.5 0.5 0.5 1.0]  GraphicVisPropType=SimpleVisualProperties
  Inertia : sm_lib/Body Elements/Inertia  InertiaType=Custom  Mass=arm.hand.mass  MassUnits=kg  CenterOfMass=[0, 0, 0]  CenterOfMassUnits=m  MomentsOfInertia=arm.hand.moment_inertia  MomentsOfInertiaUnits=kg*m^2  ProductsOfInertia=[0, 0, 0]  ProductsOfInertiaUnits=kg*m^2  GraphicType=None  MarkerShape=Inertia  MarkerSize=20  GraphicVisPropType=SimpleVisualProperties  GraphicDiffuseColor=[0.5 0.5 0.5]  GraphicSpecularColor=[0.5 0.5 0.5 1.0]  GraphicAmbientColor=[0.15 0.15 0.15 1.0]  GraphicEmissiveColor=[0.0 0.0 0.0 1.0]  GraphicShininess=75  GraphicOpacity=1.0
  Markers : Subsystem
  Mux : Mux  Inputs=3
  PS-Simulink Converter : nesl_utility/PS-Simulink Converter  PhysicalDomain=network_engine_domain  SubClassName=ps_output  LeftPortType=input  RightPortType=output  PseudoPeriodic=off  Frequencies=[]  VectorFormat=inherit  Unit=inherit  AffineConversion=off
      settings: SourceProductBaseCode=SS,PW,VE
  PS-Simulink Converter1 : nesl_utility/PS-Simulink Converter  PhysicalDomain=network_engine_domain  SubClassName=ps_output  LeftPortType=input  RightPortType=output  PseudoPeriodic=off  Frequencies=[]  VectorFormat=inherit  Unit=inherit  AffineConversion=off
      settings: SourceProductBaseCode=SS,PW,VE
  PS-Simulink Converter2 : nesl_utility/PS-Simulink Converter  PhysicalDomain=network_engine_domain  SubClassName=ps_output  LeftPortType=input  RightPortType=output  PseudoPeriodic=off  Frequencies=[]  VectorFormat=inherit  Unit=inherit  AffineConversion=off
      settings: SourceProductBaseCode=SS,PW,VE
  Reference Frame : sm_lib/Frames and Transforms/Reference Frame
  Scope : Scope
  Transform Sensor : sm_lib/Frames and Transforms/Transform Sensor  MeasurementFrame=World  SenseAngle=off  SenseAxis=off  SenseAngle1=off  SenseAngle2=off  SenseAngle3=off  SenseQ=off  SenseR=off  SenseOmegaX=off  SenseOmegaY=off  SenseOmegaZ=off  SenseOmega1=off  SenseOmega2=off  SenseOmega3=off  SenseQDot=off  SenseRDot=off  SenseAlphaX=off  SenseAlphaY=off  SenseAlphaZ=off  SenseAlpha1=off  SenseAlpha2=off  SenseAlpha3=off  SenseQDDot=off  SenseRDDot=off  SenseX=on  SenseY=on  SenseZ=on  SenseRad=off  SenseAzim=off  SenseDist=off  SenseInc=off  SenseXDot=off  SenseYDot=off  SenseZDot=off  SenseRadDot=off  SenseAzimDot=off  SenseDistDot=off  SenseIncDot=off  SenseXDDot=off  SenseYDDot=off  SenseZDDot=off  SenseRadDDot=off  SenseAzimDDot=off  SenseDistDDot=off  SenseIncDDot=off
  B_wrist : PMIOPort  Side=Left
  W : PMIOPort  Port=2  Side=Left
  wires:
  Mux/1 -> Scope/1
  PS-Simulink Converter/1 -> Mux/1  "wrist_posx"
  PS-Simulink Converter1/1 -> Mux/2  "wrist_posy"
  PS-Simulink Converter2/1 -> Mux/3  "wrist_posz"
  connections:
  B_wrist__setting/RConn1 -- Transform Sensor/RConn1 -- B_wrist/RConn1
  PS-Simulink Converter2/LConn1 -- Transform Sensor/RConn4
  PS-Simulink Converter/LConn1 -- Transform Sensor/RConn2
  PS-Simulink Converter1/LConn1 -- Transform Sensor/RConn3
  W/RConn1 -- Transform Sensor/LConn1 -- Markers/LConn1
  Hand/RConn1 -- Reference Frame/RConn1 -- Markers/LConn2 -- Inertia/RConn1 -- B_wrist__setting/LConn1

== system master_thesis_simulink/System/Human arm/RightShoulder ==
  B_shoulder__F_shoulder : sm_lib/Frames and Transforms/Rigid Transform  TranslationMethod=Cartesian  TranslationStandardOffset=0  TranslationLengthUnit=m  TranslationStandardAxis=+Z  TranslationCartesianOffset=[0 -arm.shoulder.length 0]  TranslationROffset=0  TranslationROffsetUnits=m  TranslationZOffset=0  TranslationZOffsetUnits=m  TranslationThetaOffset=0  TranslationThetaOffsetUnits=deg  RotationMethod=None  RotationAngleUnits=deg  RotationStandardAxis=+Z  RotationAngle=0.0  RotationArbitraryAxis=[0 0 1]  FollAlignAxisA=+X  BaseAlignAxisA=+Y  FollAlignAxisB=+Y  BaseAlignAxisB=+Z  RotationSequenceAxes=FollowerAxes  RotationSequence=XYX  RotationSequenceAngles=[0 0 0]  RotationSequenceAnglesUnits=deg  RotationMatrix=[1 0 0; 0 1 0; 0 0 1]
  Inertia : sm_lib/Body Elements/Inertia  InertiaType=Custom  Mass=arm.shoulder.mass  MassUnits=kg  CenterOfMass=[0 0 0]  CenterOfMassUnits=m  MomentsOfInertia=arm.shoulder.moment_inertia  MomentsOfInertiaUnits=kg*m^2  ProductsOfInertia=[0 0 0]  ProductsOfInertiaUnits=kg*m^2  GraphicType=None  MarkerShape=Inertia  MarkerSize=20  GraphicVisPropType=SimpleVisualProperties  GraphicDiffuseColor=[0.5 0.5 0.5]  GraphicSpecularColor=[0.5 0.5 0.5 1.0]  GraphicAmbientColor=[0.15 0.15 0.15 1.0]  GraphicEmissiveColor=[0.0 0.0 0.0 1.0]  GraphicShininess=75  GraphicOpacity=1.0
  Markers : Subsystem
  Mux : Mux  Inputs=3
  PS-Simulink Converter : nesl_utility/PS-Simulink Converter  PhysicalDomain=network_engine_domain  SubClassName=ps_output  LeftPortType=input  RightPortType=output  PseudoPeriodic=off  Frequencies=[]  VectorFormat=inherit  Unit=inherit  AffineConversion=off
      settings: SourceProductBaseCode=SS,PW,VE
  PS-Simulink Converter1 : nesl_utility/PS-Simulink Converter  PhysicalDomain=network_engine_domain  SubClassName=ps_output  LeftPortType=input  RightPortType=output  PseudoPeriodic=off  Frequencies=[]  VectorFormat=inherit  Unit=inherit  AffineConversion=off
      settings: SourceProductBaseCode=SS,PW,VE
  PS-Simulink Converter2 : nesl_utility/PS-Simulink Converter  PhysicalDomain=network_engine_domain  SubClassName=ps_output  LeftPortType=input  RightPortType=output  PseudoPeriodic=off  Frequencies=[]  VectorFormat=inherit  Unit=inherit  AffineConversion=off
      settings: SourceProductBaseCode=SS,PW,VE
  Reference Frame : sm_lib/Frames and Transforms/Reference Frame
  RightShoulder_rot : sm_lib/Frames and Transforms/Rigid Transform  TranslationMethod=None  TranslationStandardOffset=0  TranslationLengthUnit=m  TranslationStandardAxis=+Z  TranslationCartesianOffset=[0 0 0]  TranslationROffset=0  TranslationROffsetUnits=m  TranslationZOffset=0  TranslationZOffsetUnits=m  TranslationThetaOffset=0  TranslationThetaOffsetUnits=deg  RotationMethod=ArbitraryAxis  RotationAngleUnits=rad  RotationStandardAxis=+Z  RotationAngle=pi/2  RotationArbitraryAxis=[1 0 0]  FollAlignAxisA=+X  BaseAlignAxisA=+Y  FollAlignAxisB=+Y  BaseAlignAxisB=+Z  RotationSequenceAxes=BaseAxes  RotationSequence=XYZ  RotationSequenceAngles=[pi/2, 0, 0]  RotationSequenceAnglesUnits=rad  RotationMatrix=[1 0 0; 0 1 0; 0 0 1]
  Shoulder : sm_lib/Body Elements/Cylindrical Solid  GraphicAmbientColor=[0.15 0.15 0.15 1.0]  BasedOnType=Density  CenterOfMass=[0, 0, 0]  CenterOfMassUnits=m  GraphicDiffuseColor=[0.1, 0.1, 0.1]  CylinderLength=arm.shoulder.length  CylinderLengthUnits=m  CylinderRadius=arm.shoulder.radius  CylinderRadiusUnits=m  Density=1000  DensityUnits=kg/m^3  DoExposeReferenceFrame=on  GraphicEmissiveColor=[0.0 0.0 0.0 1.0]  ExportEntireGeometry=off  SerializedFrames=<Frames/>  MarkerShape=Sphere  MarkerSize=10  GraphicType=FromGeometry  InertiaType=CalculateFromGeometry  Mass=0  MassUnits=kg  MomentsOfInertia=[0, 0, 0]  MomentsOfInertiaUnits=kg*m^2  GraphicOpacity=1  ProductsOfInertia=[0, 0, 0]  ProductsOfInertiaUnits=kg*m^2  GraphicShininess=75  GraphicSpecularColor=[0.5 0.5 0.5 1.0]  GraphicVisPropType=SimpleVisualProperties
  Transform Sensor : sm_lib/Frames and Transforms/Transform Sensor  MeasurementFrame=World  SenseAngle=off  SenseAxis=off  SenseAngle1=off  SenseAngle2=off  SenseAngle3=off  SenseQ=off  SenseR=off  SenseOmegaX=off  SenseOmegaY=off  SenseOmegaZ=off  SenseOmega1=off  SenseOmega2=off  SenseOmega3=off  SenseQDot=off  SenseRDot=off  SenseAlphaX=off  SenseAlphaY=off  SenseAlphaZ=off  SenseAlpha1=off  SenseAlpha2=off  SenseAlpha3=off  SenseQDDot=off  SenseRDDot=off  SenseX=on  SenseY=on  SenseZ=on  SenseRad=off  SenseAzim=off  SenseDist=off  SenseInc=off  SenseXDot=off  SenseYDot=off  SenseZDot=off  SenseRadDot=off  SenseAzimDot=off  SenseDistDot=off  SenseIncDot=off  SenseXDDot=off  SenseYDDot=off  SenseZDDot=off  SenseRadDDot=off  SenseAzimDDot=off  SenseDistDDot=off  SenseIncDDot=off
  W_setting : sm_lib/Frames and Transforms/Rigid Transform  TranslationMethod=Cartesian  TranslationStandardOffset=0  TranslationLengthUnit=m  TranslationStandardAxis=+Z  TranslationCartesianOffset=[0 arm.shoulder.length/2 0]  TranslationROffset=0  TranslationROffsetUnits=m  TranslationZOffset=0  TranslationZOffsetUnits=m  TranslationThetaOffset=0  TranslationThetaOffsetUnits=deg  RotationMethod=None  RotationAngleUnits=rad  RotationStandardAxis=+Z  RotationAngle=pi/2  RotationArbitraryAxis=[1 0 0]  FollAlignAxisA=+X  BaseAlignAxisA=+Y  FollAlignAxisB=+Y  BaseAlignAxisB=+Z  RotationSequenceAxes=BaseAxes  RotationSequence=XYZ  RotationSequenceAngles=[pi/2, 0, 0]  RotationSequenceAnglesUnits=rad  RotationMatrix=[1 0 0; 0 1 0; 0 0 1]
  B_shoulder : PMIOPort  Side=Left
  F_shoulder : PMIOPort  Port=2  Side=Right
  W : PMIOPort  Port=3  Side=Left
  wires:
  PS-Simulink Converter/1 -> Mux/1  "shoulder_posx"
  PS-Simulink Converter1/1 -> Mux/2  "shoulder_posy"
  PS-Simulink Converter2/1 -> Mux/3  "shoulder_posz"
  connections:
  W_setting/RConn1 -- B_shoulder/RConn1 -- Transform Sensor/RConn1 -- B_shoulder__F_shoulder/LConn1
  F_shoulder/RConn1 -- B_shoulder__F_shoulder/RConn1
  PS-Simulink Converter2/LConn1 -- Transform Sensor/RConn4
  Transform Sensor/RConn2 -- PS-Simulink Converter/LConn1
  PS-Simulink Converter1/LConn1 -- Transform Sensor/RConn3
  RightShoulder_rot/LConn1 -- Shoulder/RConn1
  W/RConn1 -- Transform Sensor/LConn1 -- Markers/LConn1
  Inertia/RConn1 -- Reference Frame/RConn1 -- Markers/LConn2 -- RightShoulder_rot/RConn1 -- W_setting/LConn1
